simulink model "challenge_model_v2"  (R2020b)
settings: Solver=ode45  StartTime=0.0  StopTime=3  RelTol=1e-3
values from neighbouring files (symbols this model uses):
  Aq = A1q    [challenge_script_v2.m]
  Bq = [zeros(2,1) B1q zeros(2,2)]    [challenge_script_v2.m]
  enable_anti_windup = 1    [challenge_script_v2.m]
  enable_integral_action = 1    [challenge_script.m]    (also in challenge_script_v2.m)
  enable_trick = 0    [challenge_script_v2.m]
  K_ih = [K_ss_e(1)]    [challenge_script.m]    (also in challenge_script_v2.m = Ke(1))
  K_ss = [K_ss_e(2) K_ss_e(3) K_ss_e(4) K_ss_e(5)]    [challenge_script.m]    (also in challenge_script_v2.m = [Ke(2) Ke(3) Ke(4) Ke(5) Ke(6) Ke(7)])
  Kw = 0.092    [challenge_script_v2.m]
  Nu = Nxu(7)    [challenge_script_v2.m]
  Nx = [Nxu(1); Nxu(2); Nxu(3); Nxu(4); Nxu(5); Nxu(6)]    [challenge_script_v2.m]
  step_height = 50    [challenge_script.m]    (also in challenge_script_v2.m)
  step_start_time = 2    [challenge_script.m]    (also in challenge_script_v2.m = 1)
  t0 = step_start_time    (= 1)    [challenge_script_v2.m]
  t1 = t0 + 0.125    (= 1.125)    [challenge_script_v2.m]
  t2 = t1 + 0    (= 1.125)    [challenge_script_v2.m]
undefined symbols (not defined in the file or in its folder): Bb, Beq, daq, denH_w, DiscIntNeverNeededParam, drv, gbox, Jb, Jh, mld, mot, numH_w, rads2rpm, sens, tausf, Ts
libraries: simulink x6
settings Model: Creator=umberto  LastModifiedBy=irong
settings SolverCC: AlgebraicLoopSolver=LineSearch
settings DataIOCC: ReturnWorkspaceOutputs=off

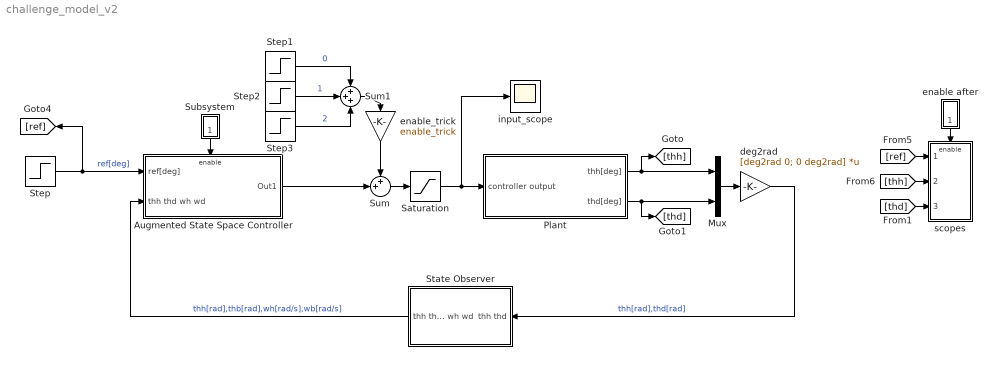
== system challenge_model_v2 ==
  Augmented State Space Controller : Subsystem
  Mux : Mux  Inputs=2
  Plant : Subsystem
  Saturation : Saturate  UpperLimit=10  LowerLimit=-10  LinearizeAsGain=off
  State Observer : Subsystem
  Step : Step  Time=step_start_time  After=step_height  SampleTime=0
  Step1 : Step  Time=t0  After=30  SampleTime=0
  Step2 : Step  Time=t1  After=-60  SampleTime=0
  Step3 : Step  Time=t2  After=30  SampleTime=0
  Subsystem : Subsystem
  Sum : Sum  Inputs=++|
  Sum1 : Sum  Inputs=+++
  deg2rad : Gain  Gain=[deg2rad 0; 0 deg2rad]  Multiplication=Matrix(K*u) (u vector)
  enable after : Subsystem
  enable_trick : Gain  Gain=enable_trick
  input_scope : Scope
  scopes : Subsystem
  wires:
  Step/1 -> Augmented State Space Controller/1(ref[deg]), [ref]  "ref[deg]"
  State Observer/1(thh thd wh wd) -> Augmented State Space Controller/2(thh thd wh wd)  "thh[rad],thb[rad],wh[rad/s],wb[rad/s]"
  Mux/1 -> deg2rad/1
  deg2rad/1 -> State Observer/1(thh thd)  "thh[rad],thd[rad]"
  Subsystem/1(0.8) -> Augmented State Space Controller/Enable
  Plant/2(thd[deg]) -> [thd], Mux/2
  Plant/1(thh[deg]) -> [thh], Mux/1
  enable after/1(1.0 s) -> scopes/Enable
  [thd] -> scopes/3(thd[deg])
  [thh] -> scopes/2(thh[deg])
  [ref] -> scopes/1(ref[deg])
  Augmented State Space Controller/1(Out1) -> Sum/2
  Sum1/1 -> enable_trick/1
  Step1/1 -> Sum1/1  "0"
  Step2/1 -> Sum1/2  "1"
  Step3/1 -> Sum1/3  "2"
  Sum/1 -> Saturation/1
  Saturation/1 -> input_scope/1, Plant/1(controller output)
  enable_trick/1 -> Sum/1

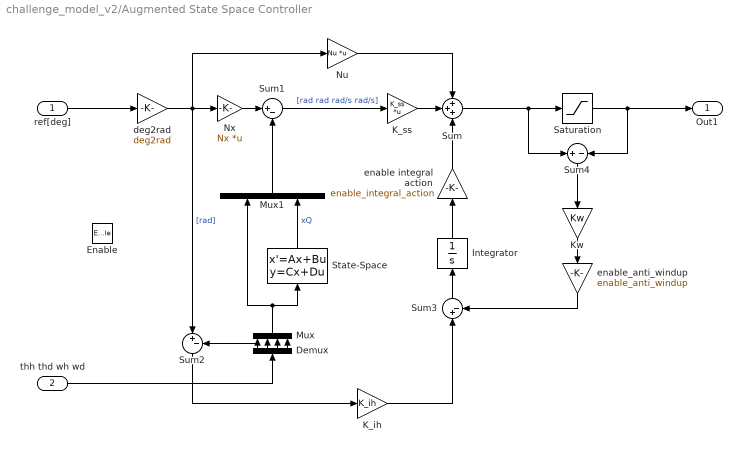
== system challenge_model_v2/Augmented State Space Controller ==
  ref[deg] : Inport
  thh thd wh wd : Inport  Port=2
  Enable : EnablePort
  Demux : Demux
  Integrator : Integrator
  K_ih : Gain  Gain=K_ih
  K_ss : Gain  Gain=K_ss  Multiplication=Matrix(K*u) (u vector)
  Kw : Gain  Gain=Kw
  Mux : Mux
  Mux1 : Mux  Inputs=2
  Nu : Gain  Gain=Nu  Multiplication=Matrix(K*u) (u vector)
  Nx : Gain  Gain=Nx  Multiplication=Matrix(K*u) (u vector)
  Saturation : Saturate  UpperLimit=10  LowerLimit=-10
  State-Space : StateSpace  A=Aq  B=Bq  C=eye(2,2)  D=zeros(2,4)  InitialCondition=0
  Sum : Sum  Inputs=+++
  Sum1 : Sum  Inputs=|+-
  Sum2 : Sum  Inputs=|+-
  Sum3 : Sum  Inputs=|+-
  Sum4 : Sum  Inputs=+|-
  deg2rad : Gain  Gain=deg2rad
  enable integral action : Gain  Gain=enable_integral_action
  enable_anti_windup : Gain  Gain=enable_anti_windup
  Out1 : Outport
  wires:
  deg2rad/1 -> Nx/1, Nu/1, Sum2/1  "[rad]"
  K_ss/1 -> Sum/2
  Nx/1 -> Sum1/1
  ref[deg]/1 -> deg2rad/1
  Nu/1 -> Sum/1
  Sum1/1 -> K_ss/1  "[rad rad rad/s rad/s]"
  Demux/1 -> Mux/1, Sum2/2
  Demux/2 -> Mux/2
  Demux/3 -> Mux/3
  Demux/4 -> Mux/4
  thh thd wh wd/1 -> Demux/1
  Sum2/1 -> K_ih/1
  enable integral action/1 -> Sum/3
  Mux/1 -> State-Space/1, Mux1/1
  State-Space/1 -> Mux1/2  "xQ"
  Mux1/1 -> Sum1/2
  Integrator/1 -> enable integral action/1
  Sum3/1 -> Integrator/1
  K_ih/1 -> Sum3/1
  Sum/1 -> Sum4/1, Saturation/1
  Saturation/1 -> Sum4/2, Out1/1
  enable_anti_windup/1 -> Sum3/2
  Kw/1 -> enable_anti_windup/1
  Sum4/1 -> Kw/1

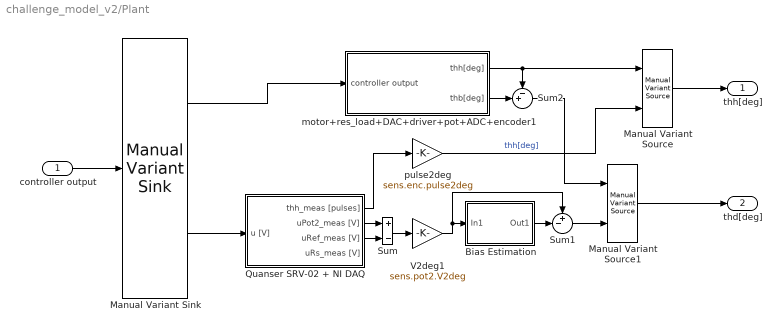
== system challenge_model_v2/Plant ==
  controller output : Inport
  Bias Estimation : Subsystem
  Manual Variant Sink : simulink/Signal Routing/Manual Variant Sink  NumChoices=2  LabelModeActiveChoice=V_2
  Manual Variant Source : simulink/Signal Routing/Manual Variant Source  NumChoices=2  LabelModeActiveChoice=V_2
  Manual Variant Source1 : simulink/Signal Routing/Manual Variant Source  NumChoices=2  LabelModeActiveChoice=V_2
  Quanser SRV-02 + NI DAQ : Subsystem  mask(Quanser SRV-02 (with resonant load) + NI DAQ){Ts=Ts, fricType=Karnopp, lockShaft=off, beamInitPos=10}
      mask prompts: Ts "NI DAQ Sample Time:"; fricType "Friction model"; lockShaft "Lock motor shaft"; beamInitPos "Beam initial position [deg]:"
      mask help: Quanser SRV-02 (with resonant load) + NI DAQ model.
      mask init:
      | %%
      | % Riccardo Antonello (riccardo.antonello@unipd.it)
      | %
      | % April 28, 2020
      | %
      | % Dept. of Information Engineering, University of Padova
      | %
      | 
      | %%  Conversion gains
      | deg2rad = pi/180;                   %   [deg]   -> [rad]
      | rad2deg = 180/pi;                   %   [rad]   -> [deg]
      | 
      | 
      | %%  Sensors data
      | 
      | %   shunt resistor
      | sens.curr.Rs = 0.5;   
      | 
      | %   Hewlett-Packard HEDS-5540#A06 optical encoder
      | sens.enc.ppr = 500*4;                                                   %   pulses per rotation
      | sens.enc.pulse2deg = 360/sens.enc.ppr;                                  %   [pulses] -> [deg]
      | sens.enc.pulse2rad = 2*pi/sens.enc.ppr;                                 %   [pulses] -> [rad]
      | sens.enc.deg2pulse = sens.enc.ppr/360;                                  %   [deg] -> [pulses]
      | sens.enc.rad2pulse = sens.enc.ppr/2/pi;                                 %   [rad] -> [pulses]
      | 
      | %   potentiometer 2 (Spectrol 357-0-0-103) - installed on hub
      | sens.pot2.range.R      = 10e3;                                          %   ohmic value range 
      | sens.pot2.range.V      = 5;                                             %   voltage range
      | sens.pot2.range.th_deg = 340;                                           %   angle range [deg]
      | sens.pot2.range.th     = sens.pot2.range.th_deg * deg2rad;              %   angle range [rad]                           
      | sens.pot2.deg2V        = sens.pot2.range.V / sens.pot2.range.th_deg;    %   sensitivity [V/deg]
      | sens.pot2.rad2V        = sens.pot2.range.V / sens.pot2.range.th;        %   sensitivity [V/rad]
      | sens.pot2.V2deg        = 1/sens.pot2.deg2V;                             %   conversion gain [V] -> [deg]
      | sens.pot2.V2rad        = 1/sens.pot2.rad2V;                             %   conversion gain [V] -> [rad]
      | sens.pot2.noise.var    = 3.5e-7;                                        %   out noise variance [V^2]
      | 
      | 
      | %%  Data acquisition board (daq) data
      | 
      | %   NI PCI-6221 DAC data
      | daq.dac.bits = 16;                                  %   resolution (bits)
      | daq.dac.fs   = 10;                                  %   full scale 
      | daq.dac.q    = 2*daq.dac.fs/(2^daq.dac.bits-1);     %	quantization
      | 
      | %   NI PCI-6221 ADC data
      | daq.adc.bits = 16;                                  %   resolution (bits)
      | daq.adc.fs   = 10;                                  %   full scale (as set in SLDRT Analog Input block)
      | daq.adc.q    = 2*daq.adc.fs/(2^daq.adc.bits-1);     %   quantization   
      | 
      | 
      | %%  Set beam initial position
      | % SRV02Handle = find_system(gcb, ...
      | %     'LookUnderMasks', 'on', ...
      | %     'FindAll', 'on', ...
      | %     'FollowLinks', 'on', ...
      | %     'SearchDepth', '1', ...
      | %     'BlockType', 'ModelReference', ...
      | %     'Name', 'Quanser SRV-02');
      | %
      | % %get_param(SRV02Handle, 'InstanceParameters')
      | % InstanceParams = get_param(SRV02Handle, 'InstanceParameters');
      | % for k = 1:length(InstanceParams)
      | %     if strcmp(InstanceParams(k).Name, 'thb0')
      | %         if lockShaft
      | %             InstanceParams(k).Value = sprintf('%f', beamInitPos);
      | %         else
      | %             InstanceParams(k).Value = sprintf('%f', 0);    
      | %         end
      | %         set_param(SRV02Handle, 'InstanceParameters', InstanceParams);
      | %         break;
      | %     end
      | % end
      | 
      | if lockShaft
      |     thb0 = beamInitPos;
      | else
      |     thb0 = 0;    
      | end
      | 
      | 
      | %%  Mask initialization
      | if lockShaft
      |     
      |     %   find Inport handle
      |     InPortHandle = find_system(gcb, ...
      |         'LookUnderMasks', 'on', ...
      |         'FindAll', 'on', ...
      |         'FollowLinks', 'on', ...
      |         'SearchDepth', '1', ...
      |         'BlockType', 'Inport', ...
      |         'Name', 'u [V]');
      |     
      |     if ~isempty(InPortHandle)
      |     
      |         %   find DAC handle
      |         DACHandle = find_system(gcb, ...
      |             'LookUnderMasks', 'on', ...
      |             'FindAll', 'on', ...
      |             'FollowLinks', 'on', ...
      |             'SearchDepth', '1', ...
      |             'BlockType', 'SubSystem', ...
      |             'Name', 'DAC');  
      | 
      |         %   remove Inport output connection   
      |         InportConn = get_param(InPortHandle, 'PortConnectivity');
      |         delete_line(gcb, InportConn.Position);
      | 
      |         %   remove Inport block
      |         delete_block(InPortHandle);
      | 
      |         %   add Constant block
      |         ConstantHandle = add_block( ...
      |             'simulink/Sources/Constant', [gcb, '/u [V]'], ...
      |             'Position', [20   -37    50   -23], ...
      |             'Value', '0');
      | 
      |         %   connect Constant to DAC block
      |         DACPortHandles = get_param(DACHandle, 'PortHandles');
      |         ConstantPortHandles = get_param(ConstantHandle, 'PortHandles');
      |         add_line(gcb, ConstantPortHandles.Outport(1), DACPortHandles.Inport(1));
      |     
      |     end
      |     
      | else
      |     
      |     %   find Constant handle
      |     ConstantHandle = find_system(gcb, ...
      |         'LookUnderMasks', 'on', ...
      |         'FindAll', 'on', ...
      |         'FollowLinks', 'on', ...
      |         'SearchDepth', '1', ...
      |         'BlockType', 'Constant', ...
      |         'Name', 'u [V]');
      |     
      |     if ~isempty(ConstantHandle)
      |     
      |         %   find DAC handle
      |         DACHandle = find_system(gcb, ...
      |             'LookUnderMasks', 'on', ...
      |             'FindAll', 'on', ...
      |             'FollowLinks', 'on', ...
      |             'SearchDepth', '1', ...
      |             'BlockType', 'SubSystem', ...
      |             'Name', 'DAC');  
      |  
      |         %   remove Constant output connection   
      |         ConstantConn = get_param(ConstantHandle, 'PortConnectivity');
      |         delete_line(gcb, ConstantConn.Position);
      | 
      |         %   remove Inport block
      |         delete_block(ConstantHandle);   
      | 
      |         %   add Inport block
      |         InportHandle = add_block( ...
      |             'simulink/Sources/In1', [gcb, '/u [V]'], ...
      |             'Position', [20   -37    50   -23], ...
      |             'Port', '1');
      | 
      |         %   connect Constant to DAC block
      |         DACPortHandles = get_param(DACHandle, 'PortHandles');
      |         InportPortHandles = get_param(InportHandle, 'PortHandles');
      |         add_line(gcb, InportPortHandles.Outport(1), DACPortHandles.Inport(1));
      |     
      |      end
      |     
      | end
      mask Help:
      | Riccardo Antonello (antonello@dei.unipd.it)
      | 
      | April 28, 2020
      | 
      | Dept. of Information Engineering, University of Padova
      mask TypeOptions fricType: Coulomb + viscous | Karnopp
      mask Callback lockShaft:
      | %   get status of check box
      | lockShaft = get_param(gcb, 'lockShaft');
      | 
      | %   get current value of MaskVisibilities property
      | maskVisibilities = get_param(gcb, 'MaskVisibilities');
      | 
      | %   set visibility of the dialog box element
      | if strcmp(lockShaft, 'on')
      |     maskVisibilities{4} = 'on';
      | else
      |     maskVisibilities{4} = 'off';
      | end
      | 
      | % Set the 'MaskVisibilities' property for each parameter in mask
      | set_param( gcb, 'MaskVisibilities', maskVisibilities);
  Sum : Sum  Inputs=+-
  Sum1 : Sum  Inputs=+-|
  Sum2 : Sum  Inputs=-+|
  V2deg1 : Gain  Gain=sens.pot2.V2deg
  motor+res_load+DAC+driver+pot+ADC+encoder1 : Subsystem
  pulse2deg : Gain  Gain=sens.enc.pulse2deg
  thh[deg] : Outport
  thd[deg] : Outport  Port=2
  wires:
  Manual Variant Source1/1 -> thd[deg]/1
  controller output/1 -> Manual Variant Sink/1
  Manual Variant Sink/1 -> motor+res_load+DAC+driver+pot+ADC+encoder1/1(controller output)
  Manual Variant Sink/2 -> Quanser SRV-02 + NI DAQ/1(u [V])
  motor+res_load+DAC+driver+pot+ADC+encoder1/1(thh[deg]) -> Sum2/1, Manual Variant Source/1
  Manual Variant Source/1 -> thh[deg]/1
  Quanser SRV-02 + NI DAQ/1(thh_meas [pulses]) -> pulse2deg/1
  Bias Estimation/1(Out1) -> Sum1/2
  Sum1/1 -> Manual Variant Source1/2
  motor+res_load+DAC+driver+pot+ADC+encoder1/2(thb[deg]) -> Sum2/2
  Sum2/1 -> Manual Variant Source1/1
  pulse2deg/1 -> Manual Variant Source/2  "thh[deg]"
  Quanser SRV-02 + NI DAQ/3(uRef_meas [V]) -> Sum/2
  Sum/1 -> V2deg1/1
  Quanser SRV-02 + NI DAQ/2(uPot2_meas [V]) -> Sum/1
  V2deg1/1 -> Sum1/1, Bias Estimation/1(In1)

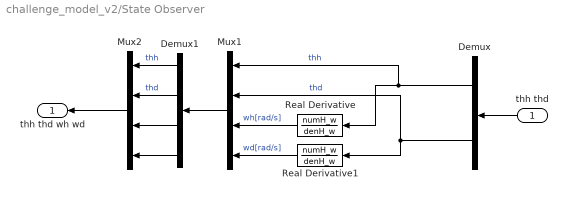
== system challenge_model_v2/State Observer ==
  thh thd : Inport
  Demux : Demux  Outputs=2
  Demux1 : Demux
  Mux1 : Mux
  Mux2 : Mux
  Real Derivative : TransferFcn  Numerator=numH_w  Denominator=denH_w
  Real Derivative1 : TransferFcn  Numerator=numH_w  Denominator=denH_w
  thh thd wh wd : Outport
  wires:
  Real Derivative/1 -> Mux1/3  "wh[rad/s]"
  Demux/1 -> Real Derivative/1, Mux1/1  "thh"
  thh thd/1 -> Demux/1
  Real Derivative1/1 -> Mux1/4  "wd[rad/s]"
  Demux/2 -> Mux1/2, Real Derivative1/1  "thd"
  Mux2/1 -> thh thd wh wd/1
  Mux1/1 -> Demux1/1
  Demux1/1 -> Mux2/1  "thh"
  Demux1/2 -> Mux2/2  "thd"
  Demux1/3 -> Mux2/3
  Demux1/4 -> Mux2/4

== system challenge_model_v2/Subsystem ==
  Clock : Clock
  Interval Test : simulink/Logic and Bit Operations/Interval Test  IntervalClosedRight=on  uplimit=inf  IntervalClosedLeft=on  lowlimit=0.8  OutDataTypeStr=boolean
  0.8 : Outport
  wires:
  Clock/1 -> Interval Test/1
  Interval Test/1 -> 0.8/1

== system challenge_model_v2/enable after ==
  Clock : Clock
  Interval Test : simulink/Logic and Bit Operations/Interval Test  IntervalClosedRight=on  uplimit=inf  IntervalClosedLeft=on  lowlimit=1  OutDataTypeStr=boolean
  1.0 s : Outport
  wires:
  Interval Test/1 -> 1.0 s/1
  Clock/1 -> Interval Test/1

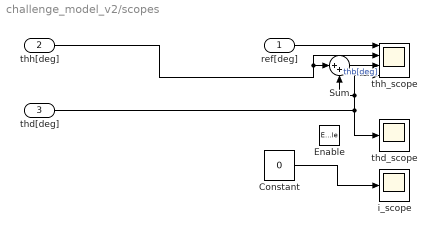
== system challenge_model_v2/scopes ==
  ref[deg] : Inport
  thh[deg] : Inport  Port=2
  thd[deg] : Inport  Port=3
  Enable : EnablePort
  Constant : Constant  Value=0
  Sum : Sum  Inputs=|++
  i_scope : Scope
  thd_scope : Scope
  thh_scope : Scope  NumInputPorts=4
  wires:
  thd[deg]/1 -> thh_scope/4, Sum/2, thd_scope/1
  Constant/1 -> i_scope/1
  thh[deg]/1 -> Sum/1, thh_scope/2
  ref[deg]/1 -> thh_scope/1
  Sum/1 -> thh_scope/3  "thb[deg]"

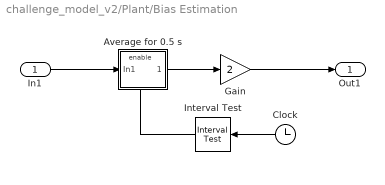
== system challenge_model_v2/Plant/Bias Estimation ==
  In1 : Inport
  Average for 0.5 s : Subsystem
  Clock : Clock
  Gain : Gain  Gain=2
  Interval Test : simulink/Logic and Bit Operations/Interval Test  IntervalClosedRight=on  uplimit=0.7  IntervalClosedLeft=on  lowlimit=0.2  OutDataTypeStr=boolean
  Out1 : Outport
  wires:
  Gain/1 -> Out1/1
  Average for 0.5 s/1(Out1) -> Gain/1
  Clock/1 -> Interval Test/1
  In1/1 -> Average for 0.5 s/1(In1)
  Interval Test/1 -> Average for 0.5 s/Enable

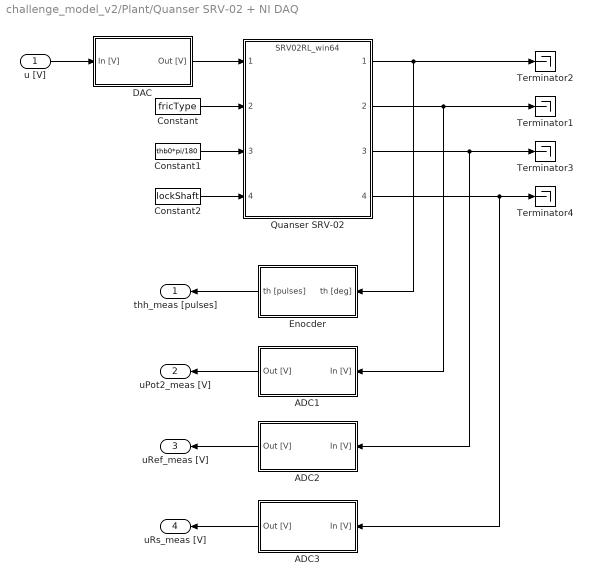
== system challenge_model_v2/Plant/Quanser SRV-02 + NI DAQ ==
  u [V] : Inport
  ADC1 : Subsystem
  ADC2 : Subsystem
  ADC3 : Subsystem
  Constant : Constant  Value=fricType
  Constant1 : Constant  Value=thb0*pi/180  SampleTime=Inf
  Constant2 : Constant  Value=lockShaft  SampleTime=Inf
  DAC : Subsystem
  Enocder : Subsystem
  Quanser SRV-02 : ModelReference  ModelNameDialog=SRV02RL_win64.slxp  ModelReferenceVersion=1.76  CopyOfModelProtected=on
  Terminator{1..4} (4 alike) : Terminator
  thh_meas [pulses] : Outport
  uPot2_meas [V] : Outport  Port=2
  uRef_meas [V] : Outport  Port=3
  uRs_meas [V] : Outport  Port=4
  wires:
  Enocder/1(th [pulses]) -> thh_meas [pulses]/1
  ADC3/1(Out [V]) -> uRs_meas [V]/1
  DAC/1(Out [V]) -> Quanser SRV-02/1
  Quanser SRV-02/2 -> ADC1/1(In [V]), Terminator1/1
  Quanser SRV-02/1 -> Terminator2/1, Enocder/1(th [deg])
  Constant/1 -> Quanser SRV-02/2
  Quanser SRV-02/3 -> ADC2/1(In [V]), Terminator3/1
  ADC1/1(Out [V]) -> uPot2_meas [V]/1
  Constant1/1 -> Quanser SRV-02/3
  Constant2/1 -> Quanser SRV-02/4
  Quanser SRV-02/4 -> ADC3/1(In [V]), Terminator4/1
  ADC2/1(Out [V]) -> uRef_meas [V]/1
  u [V]/1 -> DAC/1(In [V])

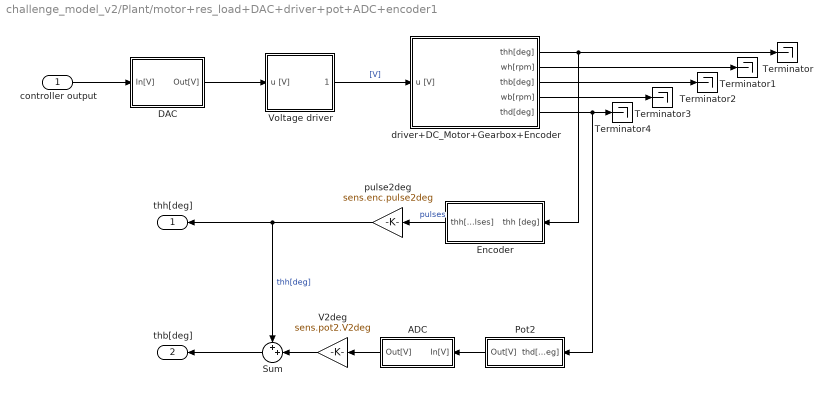
== system challenge_model_v2/Plant/motor+res_load+DAC+driver+pot+ADC+encoder1 ==
  controller output : Inport
  ADC : Subsystem
  DAC : Subsystem
  Encoder : Subsystem
  Pot2 : Subsystem
  Sum : Sum  Inputs=++|
  Terminator{,1..4} (5 alike) : Terminator
  V2deg : Gain  Gain=sens.pot2.V2deg
  Voltage driver : Subsystem
  driver+DC_Motor+Gearbox+Encoder : Subsystem
  pulse2deg : Gain  Gain=sens.enc.pulse2deg
  thh[deg] : Outport
  thb[deg] : Outport  Port=2
  wires:
  driver+DC_Motor+Gearbox+Encoder/4(wb[rpm]) -> Terminator3/1
  Voltage driver/1(udrv [V]) -> driver+DC_Motor+Gearbox+Encoder/1(u [V])  "[V]"
  pulse2deg/1 -> Sum/1, thh[deg]/1  "thh[deg]"
  driver+DC_Motor+Gearbox+Encoder/2(wh[rpm]) -> Terminator1/1
  ADC/1(Out[V]) -> V2deg/1
  V2deg/1 -> Sum/2
  DAC/1(Out[V]) -> Voltage driver/1(u [V])
  controller output/1 -> DAC/1(In[V])
  driver+DC_Motor+Gearbox+Encoder/3(thb[deg]) -> Terminator2/1
  driver+DC_Motor+Gearbox+Encoder/1(thh[deg]) -> Encoder/1("thh [deg] "), Terminator/1
  driver+DC_Motor+Gearbox+Encoder/5(thd[deg]) -> Pot2/1(thd[deg]), Terminator4/1
  Pot2/1(Out[V]) -> ADC/1(In[V])
  Sum/1 -> thb[deg]/1
  Encoder/1(thh[pulses]) -> pulse2deg/1  "pulses"

== system challenge_model_v2/Plant/Bias Estimation/Average for 0.5 s ==
  In1 : Inport
  Enable : EnablePort
  Discrete-Time Integrator : DiscreteIntegrator  SampleTime=Ts  ICPrevOutput=DiscIntNeverNeededParam  ICPrevScaledInput=DiscIntNeverNeededParam
  Out1 : Outport
  wires:
  Discrete-Time Integrator/1 -> Out1/1
  In1/1 -> Discrete-Time Integrator/1

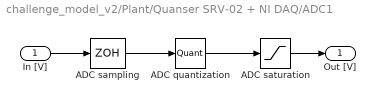
== system challenge_model_v2/Plant/Quanser SRV-02 + NI DAQ/ADC1 ==
  In [V] : Inport
  ADC quantization : Quantizer  QuantizationInterval=daq.adc.q
  ADC sampling : ZeroOrderHold  SampleTime=Ts
  ADC saturation : Saturate  UpperLimit=daq.adc.fs  LowerLimit=-daq.adc.fs
  Out [V] : Outport
  wires:
  ADC saturation/1 -> Out [V]/1
  ADC sampling/1 -> ADC quantization/1
  In [V]/1 -> ADC sampling/1
  ADC quantization/1 -> ADC saturation/1

== system challenge_model_v2/Plant/Quanser SRV-02 + NI DAQ/ADC2 ==
  In [V] : Inport
  ADC quantization : Quantizer  QuantizationInterval=daq.adc.q
  ADC sampling : ZeroOrderHold  SampleTime=Ts
  ADC saturation : Saturate  UpperLimit=daq.adc.fs  LowerLimit=-daq.adc.fs
  Out [V] : Outport
  wires:
  ADC quantization/1 -> ADC saturation/1
  In [V]/1 -> ADC sampling/1
  ADC sampling/1 -> ADC quantization/1
  ADC saturation/1 -> Out [V]/1

== system challenge_model_v2/Plant/Quanser SRV-02 + NI DAQ/ADC3 ==
  In [V] : Inport
  Quantizer : Quantizer  QuantizationInterval=daq.adc.q
  Saturation : Saturate  UpperLimit=daq.adc.fs  LowerLimit=-daq.adc.fs
  Zero-Order Hold : ZeroOrderHold  SampleTime=Ts
  Out [V] : Outport
  wires:
  Saturation/1 -> Out [V]/1
  In [V]/1 -> Zero-Order Hold/1
  Quantizer/1 -> Saturation/1
  Zero-Order Hold/1 -> Quantizer/1

== system challenge_model_v2/Plant/Quanser SRV-02 + NI DAQ/DAC ==
  In [V] : Inport
  Quantizer : Quantizer  QuantizationInterval=daq.dac.q
  Saturation : Saturate  UpperLimit=daq.dac.fs  LowerLimit=-daq.dac.fs
  Zero-Order Hold : ZeroOrderHold  SampleTime=Ts
  Out [V] : Outport
  wires:
  Quantizer/1 -> Saturation/1
  In [V]/1 -> Zero-Order Hold/1
  Zero-Order Hold/1 -> Quantizer/1
  Saturation/1 -> Out [V]/1

== system challenge_model_v2/Plant/Quanser SRV-02 + NI DAQ/Enocder ==
  th [deg] : Inport
  Quantizer : Quantizer  QuantizationInterval=sens.enc.pulse2deg
  Zero-Order Hold : ZeroOrderHold  SampleTime=Ts
  deg2pulse : Gain  Gain=sens.enc.deg2pulse
  th [pulses] : Outport
  wires:
  Quantizer/1 -> deg2pulse/1
  th [deg]/1 -> Zero-Order Hold/1
  Zero-Order Hold/1 -> Quantizer/1
  deg2pulse/1 -> th [pulses]/1

== system challenge_model_v2/Plant/motor+res_load+DAC+driver+pot+ADC+encoder1/ADC ==
  In[V] : Inport
  ADC quantization : Quantizer  QuantizationInterval=daq.adc.q
  ADC sampling : ZeroOrderHold  SampleTime=Ts
  ADC saturation : Saturate  UpperLimit=daq.adc.fs  LowerLimit=-daq.adc.fs
  Out[V] : Outport
  wires:
  ADC saturation/1 -> Out[V]/1
  ADC sampling/1 -> ADC quantization/1
  In[V]/1 -> ADC sampling/1
  ADC quantization/1 -> ADC saturation/1

== system challenge_model_v2/Plant/motor+res_load+DAC+driver+pot+ADC+encoder1/DAC ==
  In[V] : Inport
  Quantizer : Quantizer  QuantizationInterval=daq.dac.q
  Saturation : Saturate  UpperLimit=daq.dac.fs  LowerLimit=-daq.dac.fs  LinearizeAsGain=off
  Zero-Order Hold : ZeroOrderHold  SampleTime=Ts
  Out[V] : Outport
  wires:
  In[V]/1 -> Zero-Order Hold/1
  Quantizer/1 -> Saturation/1
  Zero-Order Hold/1 -> Quantizer/1
  Saturation/1 -> Out[V]/1

== system challenge_model_v2/Plant/motor+res_load+DAC+driver+pot+ADC+encoder1/Encoder ==
  "thh [deg] " : Inport
  Gain : Gain  Gain=sens.enc.ppr/360
  Quantizer : Quantizer  QuantizationInterval=sens.enc.pulse2deg
  Zero-Order Hold : ZeroOrderHold  SampleTime=Ts
  thh[pulses] : Outport
  wires:
  "thh [deg] "/1 -> Zero-Order Hold/1
  Zero-Order Hold/1 -> Quantizer/1
  Quantizer/1 -> Gain/1
  Gain/1 -> thh[pulses]/1

== system challenge_model_v2/Plant/motor+res_load+DAC+driver+pot+ADC+encoder1/Pot2 ==
  thd[deg] : Inport
  Sensor Output Noise [V] : RandomNumber  Variance=sens.pot2.noise.var  SampleTime=Ts
  Sum : Sum  Inputs=|++
  deg2V : Gain  Gain=sens.pot2.deg2V
  Out[V] : Outport
  wires:
  Sum/1 -> Out[V]/1
  Sensor Output Noise [V]/1 -> Sum/2
  deg2V/1 -> Sum/1
  thd[deg]/1 -> deg2V/1

== system challenge_model_v2/Plant/motor+res_load+DAC+driver+pot+ADC+encoder1/Voltage driver ==
  u [V] : Inport
  Saturation : Saturate  UpperLimit=drv.outmax  LowerLimit=-drv.outmax  LinearizeAsGain=off
  Transfer Fcn : TransferFcn  Numerator=[drv.dcgain]  Denominator=[drv.Tc 1]
  udrv [V] : Outport
  wires:
  u [V]/1 -> Transfer Fcn/1
  Transfer Fcn/1 -> Saturation/1
  Saturation/1 -> udrv [V]/1

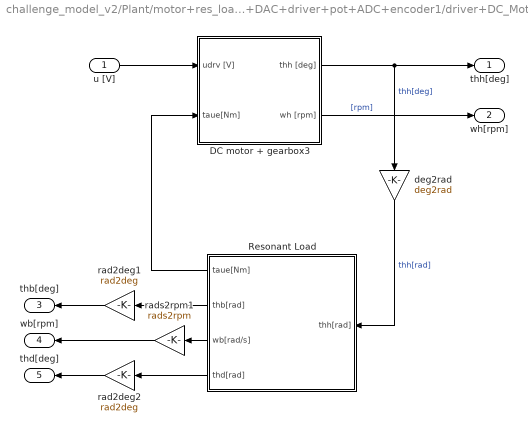
== system challenge_model_v2/Plant/motor+res_load+DAC+driver+pot+ADC+encoder1/driver+DC_Motor+Gearbox+Encoder ==
  u [V] : Inport
  DC motor + gearbox3 : Subsystem
  Resonant Load : Subsystem
  deg2rad : Gain  Gain=deg2rad
  rad2deg1 : Gain  Gain=rad2deg
  rad2deg2 : Gain  Gain=rad2deg
  rads2rpm1 : Gain  Gain=rads2rpm
  thh[deg] : Outport
  wh[rpm] : Outport  Port=2
  thb[deg] : Outport  Port=3
  wb[rpm] : Outport  Port=4
  thd[deg] : Outport  Port=5
  wires:
  rad2deg2/1 -> thd[deg]/1
  rads2rpm1/1 -> wb[rpm]/1
  rad2deg1/1 -> thb[deg]/1
  Resonant Load/4(thd[rad]) -> rad2deg2/1
  Resonant Load/3(wb[rad/s]) -> rads2rpm1/1
  Resonant Load/2(thb[rad]) -> rad2deg1/1
  Resonant Load/1(taue[Nm]) -> DC motor + gearbox3/2(taue[Nm])
  deg2rad/1 -> Resonant Load/1(thh[rad])  "thh[rad]"
  u [V]/1 -> DC motor + gearbox3/1(udrv [V])
  DC motor + gearbox3/1("thh [deg] ") -> deg2rad/1, thh[deg]/1  "thh[deg]"
  DC motor + gearbox3/2(wh [rpm]) -> wh[rpm]/1  "[rpm]"

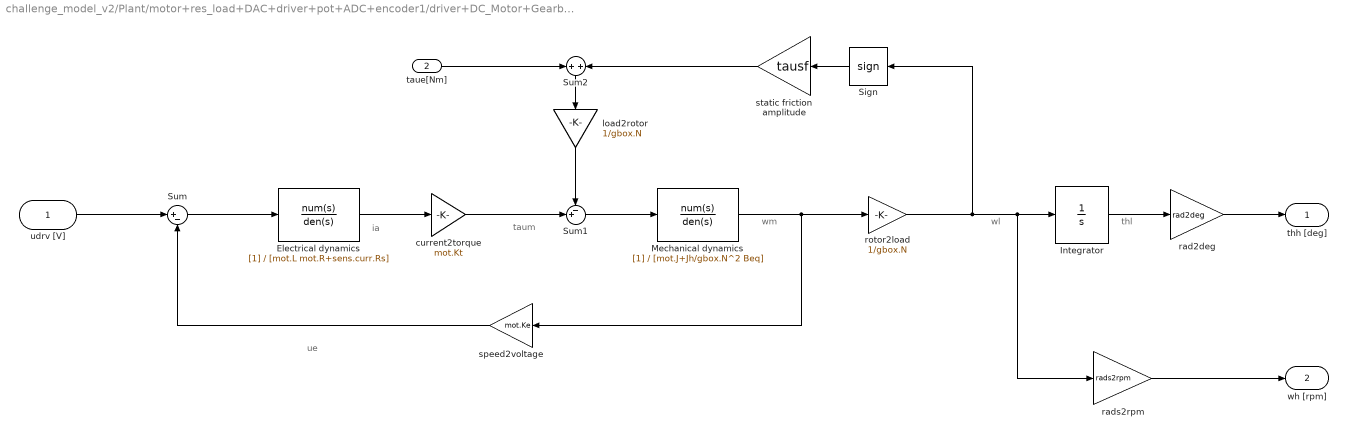
== system challenge_model_v2/Plant/motor+res_load+DAC+driver+pot+ADC+encoder1/driver+DC_Motor+Gearbox+Encoder/DC motor + gearbox3 ==
  note: ia
  note: taum
  note: ue
  note: wm
  note: wl
  note: thl
  udrv [V] : Inport
  taue[Nm] : Inport  Port=2
  Electrical dynamics : TransferFcn  Denominator=[mot.L mot.R+sens.curr.Rs]
  Integrator : Integrator
  Mechanical dynamics : TransferFcn  Denominator=[mot.J+Jh/gbox.N^2 Beq]
  Sign : Signum  ZeroCross=off
  Sum : Sum  Inputs=|+-
  Sum1 : Sum  Inputs=-+|
  Sum2 : Sum  Inputs=+|+
  current2torque : Gain  Gain=mot.Kt
  load2rotor : Gain  Gain=1/gbox.N
  rad2deg : Gain  Gain=rad2deg
  rads2rpm : Gain  Gain=rads2rpm
  rotor2load : Gain  Gain=1/gbox.N
  speed2voltage : Gain  Gain=mot.Ke
  static friction amplitude : Gain  Gain=tausf
  "thh [deg] " : Outport
  wh [rpm] : Outport  Port=2
  wires:
  taue[Nm]/1 -> Sum2/1
  static friction amplitude/1 -> Sum2/2
  Sum2/1 -> load2rotor/1
  current2torque/1 -> Sum1/2
  load2rotor/1 -> Sum1/1
  Sum1/1 -> Mechanical dynamics/1
  Integrator/1 -> rad2deg/1
  rotor2load/1 -> Integrator/1, rads2rpm/1, Sign/1
  Sum/1 -> Electrical dynamics/1
  rads2rpm/1 -> wh [rpm]/1
  Mechanical dynamics/1 -> rotor2load/1, speed2voltage/1
  rad2deg/1 -> "thh [deg] "/1
  speed2voltage/1 -> Sum/2
  Sign/1 -> static friction amplitude/1
  Electrical dynamics/1 -> current2torque/1
  udrv [V]/1 -> Sum/1

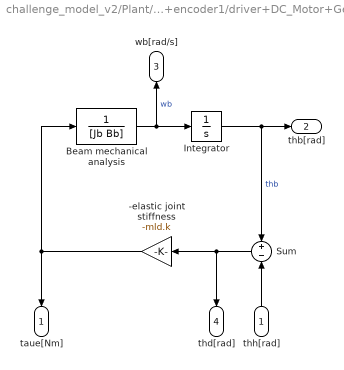
== system challenge_model_v2/Plant/motor+res_load+DAC+driver+pot+ADC+encoder1/driver+DC_Motor+Gearbox+Encoder/Resonant Load ==
  thh[rad] : Inport
  -elastic joint stiffness : Gain  Gain=-mld.k
  Beam mechanical analysis : TransferFcn  Denominator=[Jb Bb]
  Integrator : Integrator
  Sum : Sum  Inputs=+|-
  taue[Nm] : Outport
  thb[rad] : Outport  Port=2
  wb[rad/s] : Outport  Port=3
  thd[rad] : Outport  Port=4
  wires:
  Beam mechanical analysis/1 -> wb[rad/s]/1, Integrator/1  "wb"
  thh[rad]/1 -> Sum/2
  -elastic joint stiffness/1 -> taue[Nm]/1, Beam mechanical analysis/1
  Integrator/1 -> Sum/1, thb[rad]/1  "thb"
  Sum/1 -> thd[rad]/1, -elastic joint stiffness/1
